simulink model "SimEx1"  (R2023b)
settings: Solver=ode4  StartTime=0.0  StopTime=10000  FixedStep=0.1  RelTol=1e-3
values from neighbouring files (symbols this model uses):
  a = 10000    [Ex7.m]
  A = 0.01 .* [6 6 6 6 4 4 12 12 12 12]'    [Ex7.m]
  A0 = eye(3)    [Ex7.m]
  c = astroConstants(5)    [Ex7.m]
  e = 0.5    [Ex7.m]
  i = pi/6    (= 0.523598775598)    [Ex7.m]
  J = [I_x 0 0; 0 I_y 0; 0 0 I_z]    [Ex7.m]
  J_inv = inv(J)    [Ex7.m]
  jB = [0.01 0.05 0.01]' .* 1e-9    [Ex7.m]
  mu = astroConstants(13)    [Ex7.m]
  n_orb = sqrt(mu/(a^3))    [Ex7.m]
  Nb_vers = [1 0 0; 0 1 0; -1 0 0; 0 -1 0; 0 0 1; 0 0 -1; 1 0 0; -1 0 0; 1 0 0; -1 0 0]    [Ex7.m]
  om0 = [om_x0 om_y0 om_z0]    [Ex7.m]
  om_earth = 15.04 * (pi/180) * 1/3600    (= 7.29159776389e-05)    [Ex7.m]
  om_L = [om_x_L om_y_L om_z_L]'    [Ex7.m]
  R_earth = astroConstants(23)    [Ex7.m]
  rf = [10 0 0; 0 10 0; -10 0 0; 0 -10 0; 0 0 15; 0 0 -15; 0 0 45; 0 0 45; 0 0 -45; 0 0 -45] .* 1e-2    [Ex7.m]
  rho_d = 0.1 * ones(10,1)    [Ex7.m]
  rho_s = [0.5 0.5 0.5 0.5 0.5 0.5 0.1 0.1 0.1 0.1]'    [Ex7.m]
  Rs = astroConstants(3)    [Ex7.m]
libraries: matrix_library x6
settings Model: Creator=Stefano  LastModifiedBy=Stefano

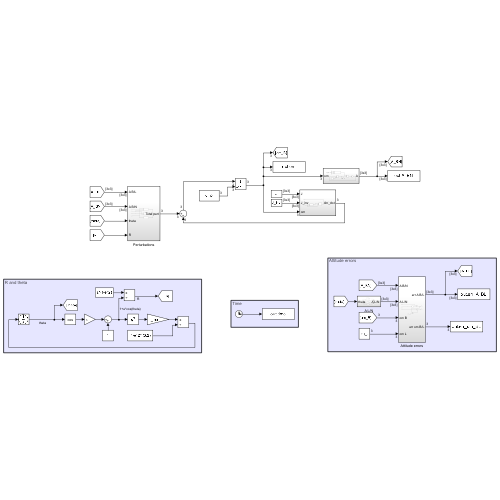
[thumbnail: Simulink's stored preview of the top-level diagram]
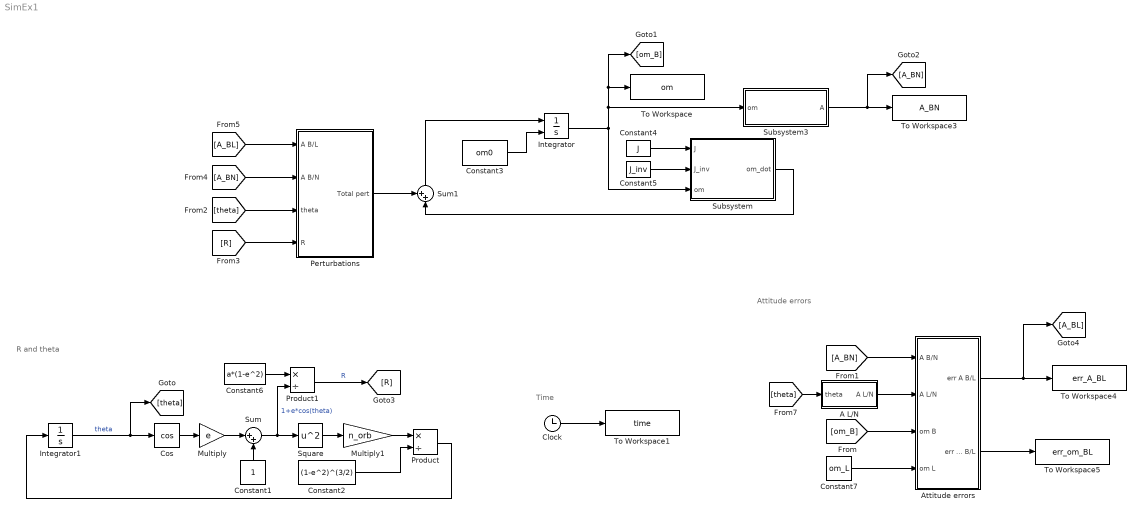
== system SimEx1 ==
  note: R and theta
  note: Time
  note: Attitude errors
  A L/N : Subsystem
  Attitude errors : Subsystem
  Clock : Clock
  Constant1 : Constant
  Constant2 : Constant  Value=(1-e^2)^(3/2)
  Constant3 : Constant  Value=om0
  Constant4 : Constant  Value=J
  Constant5 : Constant  Value=J_inv
  Constant6 : Constant  Value=a*(1-e^2)
  Constant7 : Constant  Value=om_L
  Cos : Trigonometry  Operator=cos
  Integrator : Integrator  InitialConditionSource=external
  Integrator1 : Integrator  WrapState=on  WrappedStateUpperValue=2*pi  WrappedStateLowerValue=0
  Multiply : Gain  Gain=e
  Multiply1 : Gain  Gain=n_orb
  Perturbations : Subsystem
  Product : Product  Inputs=*/
  Product1 : Product  Inputs=*/
  Square : Math  Operator=square
  Subsystem : Subsystem
  Subsystem3 : Subsystem
  Sum : Sum  Inputs=|++
  Sum1 : Sum  Inputs=++|
  To Workspace : ToWorkspace  VariableName=om  SampleTime=-1
  To Workspace1 : ToWorkspace  VariableName=time  SampleTime=-1
  To Workspace3 : ToWorkspace  VariableName=A_BN  SampleTime=-1
  To Workspace4 : ToWorkspace  VariableName=err_A_BL  SampleTime=-1
  To Workspace5 : ToWorkspace  VariableName=err_om_BL  SampleTime=-1
  wires:
  Constant3/1 -> Integrator/2
  Constant4/1 -> Subsystem/1(J)
  Constant5/1 -> Subsystem/2(J_inv)
  Integrator/1 -> Subsystem3/1(om), [om_B], To Workspace/1, Subsystem/3(om)
  Subsystem/1(om_dot) -> Sum1/2
  Clock/1 -> To Workspace1/1
  Subsystem3/1(A) -> [A_BN], To Workspace3/1
  Constant7/1 -> Attitude errors/4(om L)
  [om_B] -> Attitude errors/3(om B)
  [A_BN] -> Attitude errors/1(A B/N)
  Attitude errors/1(err A B/L) -> [A_BL], To Workspace4/1
  Attitude errors/2(err om B/L) -> To Workspace5/1
  [theta] -> A L/N/1(theta)
  Integrator1/1 -> [theta], Cos/1  "theta"
  Cos/1 -> Multiply/1
  Constant1/1 -> Sum/2
  Multiply/1 -> Sum/1
  Sum/1 -> Square/1, Product1/2  "1+e*cos(theta)"
  Square/1 -> Multiply1/1
  Multiply1/1 -> Product/1
  Constant2/1 -> Product/2
  Product/1 -> Integrator1/1
  Constant6/1 -> Product1/1
  Sum1/1 -> Integrator/1
  [A_BL] -> Perturbations/1(A B/L)
  Perturbations/1(Total pert) -> Sum1/1
  Product1/1 -> [R]  "R"
  [theta] -> Perturbations/3(theta)
  [R] -> Perturbations/4(R)
  [A_BN] -> Perturbations/2(A B/N)
  A L/N/1(A L/N) -> Attitude errors/2(A L/N)

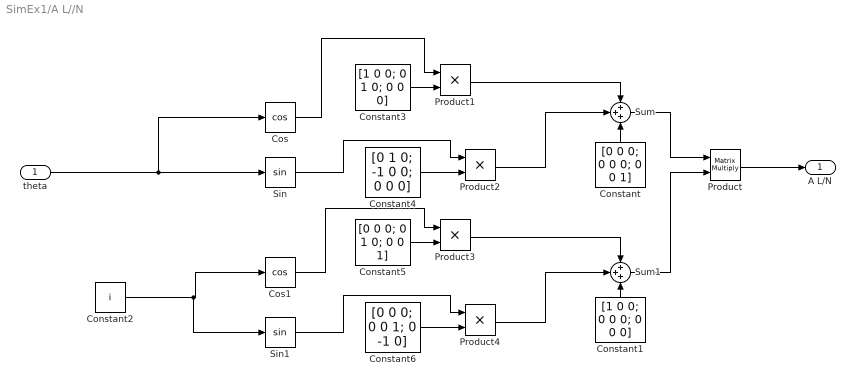
== system SimEx1/A L//N ==
  theta : Inport
  Constant : Constant  Value=[0 0 0; 0 0 0; 0 0 1]
  Constant1 : Constant  Value=[1 0 0; 0 0 0; 0 0 0]
  Constant2 : Constant  Value=i
  Constant3 : Constant  Value=[1 0 0; 0 1 0; 0 0 0]
  Constant4 : Constant  Value=[0 1 0; -1 0 0; 0 0 0]
  Constant5 : Constant  Value=[0 0 0; 0 1 0; 0 0 1]
  Constant6 : Constant  Value=[0 0 0; 0 0 1; 0 -1 0]
  Cos : Trigonometry  Operator=cos
  Cos1 : Trigonometry  Operator=cos
  Product : Product  Multiplication=Matrix(*)
  Product{1..4} (4 alike) : Product
  Sin : Trigonometry
  Sin1 : Trigonometry
  Sum : Sum  Inputs=+++
  Sum1 : Sum  Inputs=+++
  A L/N : Outport
  wires:
  theta/1 -> Cos/1, Sin/1
  Product/1 -> A L/N/1
  Sum/1 -> Product/1
  Sum1/1 -> Product/2
  Constant1/1 -> Sum1/3
  Constant/1 -> Sum/3
  Constant2/1 -> Sin1/1, Cos1/1
  Constant3/1 -> Product1/2
  Cos/1 -> Product1/1
  Constant4/1 -> Product2/2
  Product1/1 -> Sum/1
  Product2/1 -> Sum/2
  Sin/1 -> Product2/1
  Sin1/1 -> Product4/1
  Product4/1 -> Sum1/2
  Constant5/1 -> Product3/2
  Cos1/1 -> Product3/1
  Product3/1 -> Sum1/1
  Constant6/1 -> Product4/2

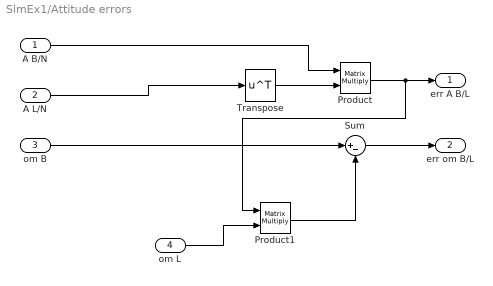
== system SimEx1/Attitude errors ==
  A B/N : Inport
  A L/N : Inport  Port=2
  om B : Inport  Port=3
  om L : Inport  Port=4
  Product : Product  Multiplication=Matrix(*)
  Product1 : Product  Multiplication=Matrix(*)
  Sum : Sum  Inputs=|+-
  Transpose : Math  Operator=transpose
  err A B/L : Outport
  err om B/L : Outport  Port=2
  wires:
  Product/1 -> Product1/1, err A B/L/1
  Transpose/1 -> Product/2
  A B/N/1 -> Product/1
  A L/N/1 -> Transpose/1
  Sum/1 -> err om B/L/1
  om B/1 -> Sum/1
  om L/1 -> Product1/2
  Product1/1 -> Sum/2

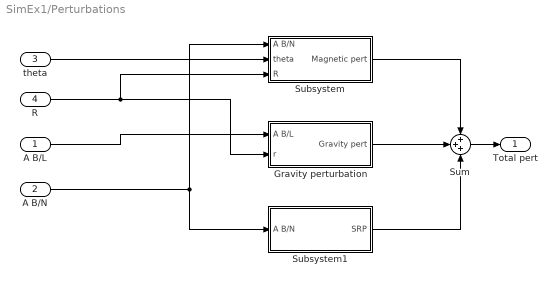
== system SimEx1/Perturbations ==
  A B/L : Inport
  A B/N : Inport  Port=2
  theta : Inport  Port=3
  R : Inport  Port=4
  Gravity perturbation : Subsystem
  Subsystem : Subsystem
  Subsystem1 : Subsystem
  Sum : Sum  Inputs=+++
  Total pert : Outport
  wires:
  Sum/1 -> Total pert/1
  Gravity perturbation/1(Gravity pert) -> Sum/2
  A B/L/1 -> Gravity perturbation/1(A B/L)
  A B/N/1 -> Subsystem/1(A B/N), Subsystem1/1(A B/N)
  theta/1 -> Subsystem/2(theta)
  R/1 -> Gravity perturbation/2(r), Subsystem/3(R)
  Subsystem/1(Magnetic pert) -> Sum/1
  Subsystem1/1(SRP) -> Sum/3

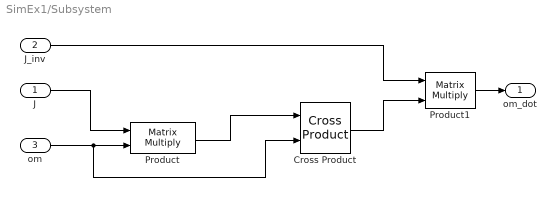
== system SimEx1/Subsystem ==
  J : Inport
  J_inv : Inport  Port=2
  om : Inport  Port=3
  Cross Product : matrix_library/Cross Product
  Product : Product  Multiplication=Matrix(*)
  Product1 : Product  Multiplication=Matrix(*)
  om_dot : Outport
  wires:
  J/1 -> Product/1
  om/1 -> Cross Product/2, Product/2
  Product/1 -> Cross Product/1
  J_inv/1 -> Product1/1
  Cross Product/1 -> Product1/2
  Product1/1 -> om_dot/1

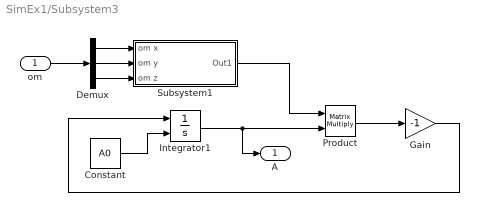
== system SimEx1/Subsystem3 ==
  om : Inport
  Constant : Constant  Value=A0
  Demux : Demux  Outputs=3
  Gain : Gain  Gain=-1
  Integrator1 : Integrator  InitialConditionSource=external
  Product : Product  Multiplication=Matrix(*)
  Subsystem1 : Subsystem
  A : Outport
  wires:
  Integrator1/1 -> A/1, Product/2
  Subsystem1/1(Out1) -> Product/1
  Demux/1 -> Subsystem1/1(om x)
  Demux/2 -> Subsystem1/2(om y)
  Product/1 -> Gain/1
  Demux/3 -> Subsystem1/3(om z)
  Constant/1 -> Integrator1/2
  Gain/1 -> Integrator1/1
  om/1 -> Demux/1

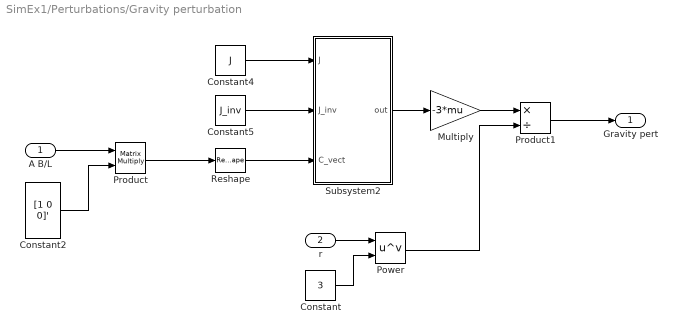
== system SimEx1/Perturbations/Gravity perturbation ==
  A B/L : Inport
  r : Inport  Port=2
  Constant : Constant  Value=3
  Constant2 : Constant  Value=[1 0 0]'  VectorParams1D=off
  Constant4 : Constant  Value=J
  Constant5 : Constant  Value=J_inv
  Multiply : Gain  Gain=-3*mu
  Power : Math  Operator=pow
  Product : Product  Multiplication=Matrix(*)
  Product1 : Product  Inputs=*/
  Reshape : Reshape
  Subsystem2 : Subsystem
  Gravity pert : Outport
  wires:
  Constant4/1 -> Subsystem2/1(J)
  Constant5/1 -> Subsystem2/2(J_inv)
  Constant2/1 -> Product/2
  Subsystem2/1(out) -> Multiply/1
  Product/1 -> Reshape/1
  Reshape/1 -> Subsystem2/3(C_vect)
  A B/L/1 -> Product/1
  Multiply/1 -> Product1/1
  Product1/1 -> Gravity pert/1
  Constant/1 -> Power/2
  r/1 -> Power/1
  Power/1 -> Product1/2

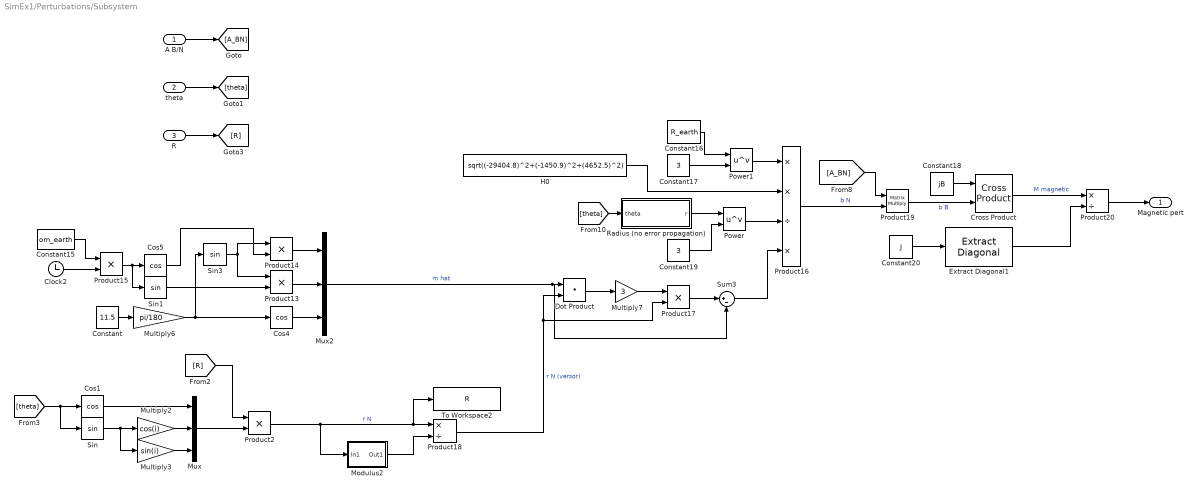
== system SimEx1/Perturbations/Subsystem ==
  A B/N : Inport
  theta : Inport  Port=2
  R : Inport  Port=3
  Clock2 : Clock
  Constant : Constant  Value=11.5
  Constant15 : Constant  Value=om_earth
  Constant16 : Constant  Value=R_earth
  Constant17 : Constant  Value=3
  Constant18 : Constant  Value=jB
  Constant19 : Constant  Value=3
  Constant20 : Constant  Value=J
  Cos1 : Trigonometry  Operator=cos
  Cos4 : Trigonometry  Operator=cos
  Cos5 : Trigonometry  Operator=cos
  Cross Product : matrix_library/Cross Product
  Dot Product : DotProduct  OutDataTypeStr=Inherit: Inherit via internal rule
  Extract Diagonal1 : matrix_library/Extract Diagonal
      settings: LibrarySourceBlock=|
      | simulink/Matrix
      | Operations/Extract Diagonal
  H0 : Constant  Value=sqrt((-29404.8)^2+(-1450.9)^2+(4652.5)^2)
  Modulus2 : Subsystem
  Multiply2 : Gain  Gain=cos(i)
  Multiply3 : Gain  Gain=sin(i)
  Multiply6 : Gain  Gain=pi/180
  Multiply7 : Gain  Gain=3
  Mux : Mux  Inputs=3
  Mux2 : Mux  Inputs=3
  Power : Math  Operator=pow
  Power1 : Math  Operator=pow
  Product{2,13..15,17} (5 alike) : Product
  Product16 : Product  Inputs=**/*
  Product18 : Product  Inputs=*/
  Product19 : Product  Multiplication=Matrix(*)
  Product20 : Product  Inputs=*/
  Radius (no error propagation) : Subsystem
  Sin : Trigonometry
  Sin1 : Trigonometry
  Sin3 : Trigonometry
  Sum3 : Sum  Inputs=|+-
  To Workspace2 : ToWorkspace  VariableName=R  SampleTime=-1
  Magnetic pert : Outport
  wires:
  [R] -> Product2/1
  Power1/1 -> Product16/1
  Constant17/1 -> Power1/2
  Multiply7/1 -> Product17/1
  Product13/1 -> Mux2/2
  H0/1 -> Product16/2
  Constant15/1 -> Product15/1
  Cos1/1 -> Mux/1
  Constant/1 -> Multiply6/1
  Multiply3/1 -> Mux/3
  Cos4/1 -> Mux2/3
  Product14/1 -> Mux2/1
  Sin3/1 -> Product14/1, Product13/1
  Product18/1 -> Dot Product/2, Product17/2  "r N (versor)"
  Multiply6/1 -> Cos4/1, Sin3/1
  Mux/1 -> Product2/2
  Extract Diagonal1/1 -> Product20/2
  [theta] -> Sin/1, Cos1/1
  Product19/1 -> Cross Product/2  "b B"
  Power/1 -> Product16/3
  Cross Product/1 -> Product20/1  "M magnetic"
  Clock2/1 -> Product15/2
  Constant20/1 -> Extract Diagonal1/1
  Product20/1 -> Magnetic pert/1
  Product15/1 -> Sin1/1, Cos5/1
  Constant16/1 -> Power1/1
  Sum3/1 -> Product16/4
  Product17/1 -> Sum3/1
  Sin/1 -> Multiply3/1, Multiply2/1
  Dot Product/1 -> Multiply7/1
  Modulus2/1(Out1) -> Product18/2
  [A_BN] -> Product19/1
  Mux2/1 -> Dot Product/1, Sum3/2  "m hat"
  Multiply2/1 -> Mux/2
  Product16/1 -> Product19/2  "b N"
  Constant18/1 -> Cross Product/1
  Product2/1 -> To Workspace2/1, Product18/1, Modulus2/1(In1)  "r N"
  Constant19/1 -> Power/2
  A B/N/1 -> [A_BN]
  theta/1 -> [theta]
  R/1 -> [R]
  Radius (no error propagation)/1(r) -> Power/1
  [theta] -> Radius (no error propagation)/1(theta)
  Cos5/1 -> Product14/2
  Sin1/1 -> Product13/2

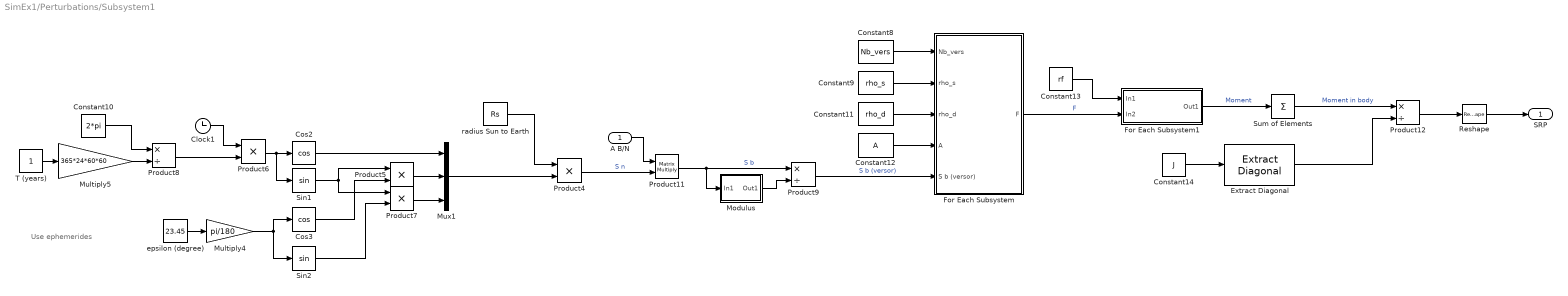
== system SimEx1/Perturbations/Subsystem1 ==
  note: Use ephemerides
  A B/N : Inport
  Clock1 : Clock
  Constant10 : Constant  Value=2*pi
  Constant11 : Constant  Value=rho_d
  Constant12 : Constant  Value=A
  Constant13 : Constant  Value=rf
  Constant14 : Constant  Value=J
  Constant8 : Constant  Value=Nb_vers
  Constant9 : Constant  Value=rho_s
  Cos2 : Trigonometry  Operator=cos
  Cos3 : Trigonometry  Operator=cos
  Extract Diagonal : matrix_library/Extract Diagonal
      settings: LibrarySourceBlock=|
      | simulink/Matrix
      | Operations/Extract Diagonal
  For Each Subsystem : Subsystem  TreatAsAtomicUnit=on
  For Each Subsystem1 : Subsystem  TreatAsAtomicUnit=on
  Modulus : Subsystem
  Multiply4 : Gain  Gain=pi/180
  Multiply5 : Gain  Gain=365*24*60*60
  Mux1 : Mux  Inputs=3
  Product11 : Product  Multiplication=Matrix(*)
  Product12 : Product  Inputs=*/
  Product{4..7} (4 alike) : Product
  Product8 : Product  Inputs=*/
  Product9 : Product  Inputs=*/
  Reshape : Reshape
  Sin1 : Trigonometry
  Sin2 : Trigonometry
  Sum of Elements : Sum  Inputs=+  CollapseMode=Specified dimension
  T (years) : Constant
  epsilon (degree) : Constant  Value=23.45
  radius Sun to Earth : Constant  Value=Rs
  SRP : Outport
  wires:
  Reshape/1 -> SRP/1
  Cos2/1 -> Mux1/1
  For Each Subsystem1/1(Out1) -> Sum of Elements/1  "Moment"
  Modulus/1(Out1) -> Product9/2
  Sum of Elements/1 -> Product12/1  "Moment in body"
  Product11/1 -> Modulus/1(In1), Product9/1  "S b"
  For Each Subsystem/1(F) -> For Each Subsystem1/2(In2)  "F"
  Constant8/1 -> For Each Subsystem/1(Nb_vers)
  Constant11/1 -> For Each Subsystem/3(rho_d)
  Constant10/1 -> Product8/1
  A B/N/1 -> Product11/1
  Product9/1 -> For Each Subsystem/5(S b (versor))  "S b (versor)"
  Multiply4/1 -> Sin2/1, Cos3/1
  Cos3/1 -> Product5/2
  Product8/1 -> Product6/2
  Multiply5/1 -> Product8/2
  Sin2/1 -> Product7/2
  Product5/1 -> Mux1/2
  Mux1/1 -> Product4/2
  Product7/1 -> Mux1/3
  epsilon (degree)/1 -> Multiply4/1
  radius Sun to Earth/1 -> Product4/1
  Sin1/1 -> Product5/1, Product7/1
  Product6/1 -> Cos2/1, Sin1/1
  Constant14/1 -> Extract Diagonal/1
  T (years)/1 -> Multiply5/1
  Product12/1 -> Reshape/1
  Constant13/1 -> For Each Subsystem1/1(In1)
  Product4/1 -> Product11/2  "S n"
  Constant9/1 -> For Each Subsystem/2(rho_s)
  Constant12/1 -> For Each Subsystem/4(A)
  Extract Diagonal/1 -> Product12/2
  Clock1/1 -> Product6/1

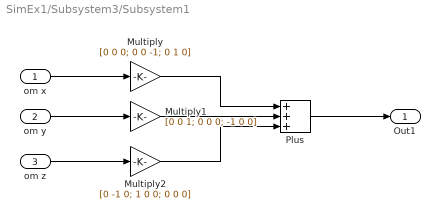
== system SimEx1/Subsystem3/Subsystem1 ==
  om x : Inport
  om y : Inport  Port=2
  om z : Inport  Port=3
  Multiply : Gain  Gain=[0 0 0; 0 0 -1; 0 1 0]
  Multiply1 : Gain  Gain=[0 0 1; 0 0 0; -1 0 0]
  Multiply2 : Gain  Gain=[0 -1 0; 1 0 0; 0 0 0]
  Plus : Sum  Inputs=+++
  Out1 : Outport
  wires:
  om x/1 -> Multiply/1
  Plus/1 -> Out1/1
  Multiply/1 -> Plus/1
  om y/1 -> Multiply1/1
  om z/1 -> Multiply2/1
  Multiply1/1 -> Plus/2
  Multiply2/1 -> Plus/3

== system SimEx1/Perturbations/Gravity perturbation/Subsystem2 ==
  J : Inport
  J_inv : Inport  Port=2
  C_vect : Inport  Port=3
  Cross Product : matrix_library/Cross Product
  Product : Product  Multiplication=Matrix(*)
  Product1 : Product  Multiplication=Matrix(*)
  out : Outport
  wires:
  J/1 -> Product/1
  C_vect/1 -> Cross Product/2, Product/2
  Product/1 -> Cross Product/1
  J_inv/1 -> Product1/1
  Cross Product/1 -> Product1/2
  Product1/1 -> out/1

== system SimEx1/Perturbations/Subsystem/Modulus2 ==
  In1 : Inport
  Dot Product : DotProduct  OutDataTypeStr=Inherit: Inherit via internal rule
  Sqrt : Sqrt
  Out1 : Outport
  wires:
  In1/1 -> Dot Product/2, Dot Product/1
  Dot Product/1 -> Sqrt/1
  Sqrt/1 -> Out1/1

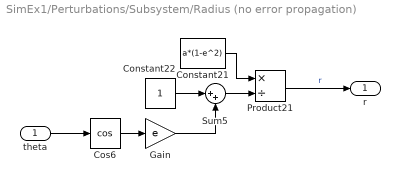
== system SimEx1/Perturbations/Subsystem/Radius (no error propagation) ==
  theta : Inport
  Constant21 : Constant  Value=a*(1-e^2)
  Constant22 : Constant
  Cos6 : Trigonometry  Operator=cos
  Gain : Gain  Gain=e
  Product21 : Product  Inputs=*/
  Sum5 : Sum  Inputs=|++
  r : Outport
  wires:
  Gain/1 -> Sum5/2
  Cos6/1 -> Gain/1
  theta/1 -> Cos6/1
  Constant21/1 -> Product21/1
  Constant22/1 -> Sum5/1
  Sum5/1 -> Product21/2
  Product21/1 -> r/1  "r"

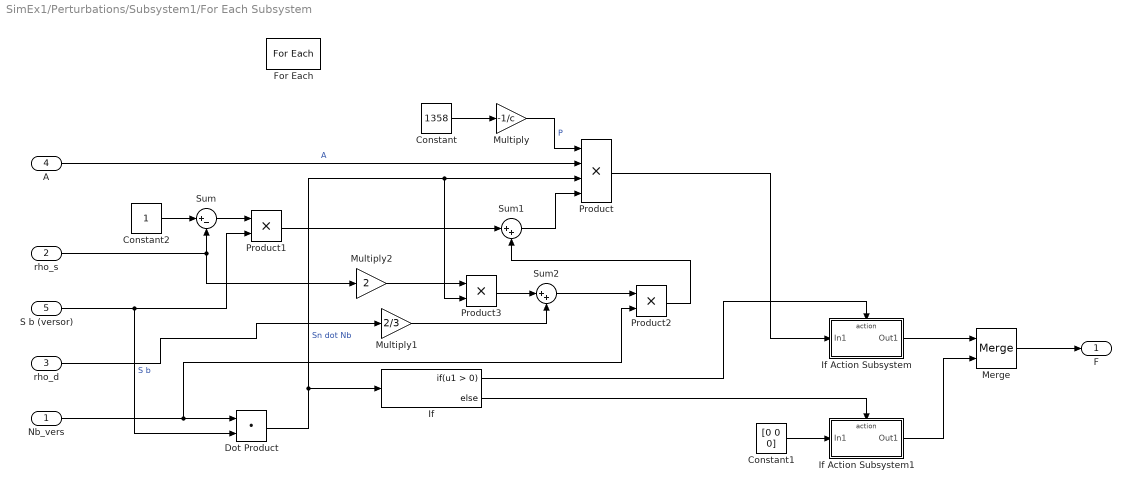
== system SimEx1/Perturbations/Subsystem1/For Each Subsystem ==
  Nb_vers : Inport  Partition=on  PartitionDimension=1  PartitionWidth=1  PartitionOffset=0
  rho_s : Inport  Port=2  Partition=on  PartitionDimension=1  PartitionWidth=1  PartitionOffset=0
  rho_d : Inport  Port=3  Partition=on  PartitionDimension=1  PartitionWidth=1  PartitionOffset=0
  A : Inport  Port=4  Partition=on  PartitionDimension=1  PartitionWidth=1  PartitionOffset=0
  S b (versor) : Inport  Port=5
  Constant : Constant  Value=1358
  Constant1 : Constant  Value=[0 0 0]
  Constant2 : Constant
  Dot Product : DotProduct  OutDataTypeStr=Inherit: Inherit via internal rule
  For Each : ForEach  DisableCoverage=on
  If : If
  If Action Subsystem : Subsystem  TreatAsAtomicUnit=on
  If Action Subsystem1 : Subsystem  TreatAsAtomicUnit=on
  Merge : Merge
  Multiply : Gain  Gain=-1/c
  Multiply1 : Gain  Gain=2/3
  Multiply2 : Gain  Gain=2
  Product : Product  Inputs=4
  Product1 : Product
  Product2 : Product
  Product3 : Product
  Sum : Sum  Inputs=|+-
  Sum1 : Sum  Inputs=|++
  Sum2 : Sum  Inputs=|++
  F : Outport  ConcatenationDimension=1
  wires:
  Dot Product/1 -> Product3/2, Product/3, If/1  "Sn dot Nb"
  If/2 -> If Action Subsystem1/Action
  If/1 -> If Action Subsystem/Action
  Constant/1 -> Multiply/1
  Multiply/1 -> Product/1  "P"
  Merge/1 -> F/1
  If Action Subsystem/1(Out1) -> Merge/1
  If Action Subsystem1/1(Out1) -> Merge/2
  Constant1/1 -> If Action Subsystem1/1(In1)
  Product/1 -> If Action Subsystem/1(In1)
  Constant2/1 -> Sum/1
  rho_s/1 -> Multiply2/1, Sum/2
  Sum/1 -> Product1/1
  Product1/1 -> Sum1/1
  Sum1/1 -> Product/4
  Product2/1 -> Sum1/2
  Sum2/1 -> Product2/1
  Multiply1/1 -> Sum2/2
  rho_d/1 -> Multiply1/1
  Product3/1 -> Sum2/1
  Multiply2/1 -> Product3/1
  Nb_vers/1 -> Product2/2, Dot Product/1
  A/1 -> Product/2  "A"
  S b (versor)/1 -> Dot Product/2, Product1/2  "S b"

== system SimEx1/Perturbations/Subsystem1/For Each Subsystem1 ==
  In1 : Inport  Partition=on  PartitionDimension=1  PartitionWidth=1  PartitionOffset=0
  In2 : Inport  Port=2  Partition=on  PartitionDimension=1  PartitionWidth=1  PartitionOffset=0
  Cross Product : matrix_library/Cross Product
  For Each : ForEach  DisableCoverage=on
  Out1 : Outport  ConcatenationDimension=1
  wires:
  In1/1 -> Cross Product/1
  In2/1 -> Cross Product/2
  Cross Product/1 -> Out1/1

== system SimEx1/Perturbations/Subsystem1/Modulus ==
  In1 : Inport
  Dot Product : DotProduct  OutDataTypeStr=Inherit: Inherit via internal rule
  Sqrt : Sqrt
  Out1 : Outport
  wires:
  In1/1 -> Dot Product/2, Dot Product/1
  Dot Product/1 -> Sqrt/1
  Sqrt/1 -> Out1/1

== system SimEx1/Perturbations/Subsystem1/For Each Subsystem/If Action Subsystem ==
  In1 : Inport
  Action Port : ActionPort  ActionPortLabel=if(u1 > 0)
  Out1 : Outport
  wires:
  In1/1 -> Out1/1

== system SimEx1/Perturbations/Subsystem1/For Each Subsystem/If Action Subsystem1 ==
  In1 : Inport
  Action Port : ActionPort  ActionPortLabel=else
  Out1 : Outport
  wires:
  In1/1 -> Out1/1
